simulink subsystem "Out_of_Plane_Model"  (R2025b)
settings: Solver=VariableStepAuto  StartTime=0.0  StopTime=10.0  RelTol=1e-3
undefined symbols (not defined in the file): AeroLiftCff, AeroLongDrgCff, AeroMotoEffctArea, AeroPitchMomentCff, AeroPitchMomentLngth, AeroRltWindAngVect, AeroSideFrcCff, AeroYawMomentCff, aMode, BrkFrntBrkActrBore, BrkFrntBrkActrPrsBpt, BrkFrntBrkPadMeanRadius, BrkFrntBrkTrqTbl, BrkFrntIntrnRadius, BrkFrntKinFricCff, BrkFrntPadNum, BrkFrntShoePinToDrumCntrDst, BrkFrntShoePinToFrcAppDst, BrkFrntShoePinToPadEndAng, BrkFrntShoePinToPadStartAng, BrkFrntStcFricCff, BrkFrntWhlSpdBpt, BrkRearBrkActrBore, BrkRearBrkActrPrsBpt, BrkRearBrkPadMeanRadius, BrkRearBrkTrqTbl, BrkRearIntrnRadius, BrkRearKinFricCff, BrkRearPadNum, BrkRearShoePinToDrumCntrDst, BrkRearShoePinToFrcAppDst, BrkRearShoePinToPadEndAng, BrkRearShoePinToPadStartAng, BrkRearStcFricCff, BrkRearWhlSpdBpt, CpRrVx0, CpRrVy0, CpRrY0, EnvAbsPrs, EnvAirTemp, FrkFrL0, FrmAng0, g, GasCnst, InitFrkLngth, InitMainFrmPitchAng, InitRearArmPitchAng, InitRearCntctPtchLatVel, InitRearCntctPtchLongVel, InitRearCntctPtchZ, InitYawAng, MotoFrmLngth, MotoFrmMass, MotoGrvty, MotoLatOfst, MotoLongOfst, MotoLowrFrntFrkMass, MotoPtchOfst, MotoRearArmLngth, MotoRearArmMass ... (+28)
libraries: sm_lib x309, nesl_utility_internal x158, nesl_utility x7, autolibsharedcoupling x6, vehdynlibtire x6, sharedtransform x4, shared6dof x1, matrix_library x1, vehdynlibeomcommon x1
(part 10 of 10)

== system Out_of_Plane_Model/Chassis, Tires, and Areo/Tire/Front Tire/Linear Front Simscape Tire/Brake model/MW Brake/Brakes/No Brake ==
  BrkPrs : Inport
  Omega : Inport  Port=2
  Ground : Ground
  Terminator : Terminator
  Terminator1 : Terminator
  MyBrk : Outport  VectorParamsAs1DForOutWhenUnconnected=off
  wires:
  BrkPrs/1 -> Terminator/1
  Ground/1 -> MyBrk/1
  Omega/1 -> Terminator1/1

== system Out_of_Plane_Model/Chassis, Tires, and Areo/Tire/Front Tire/Linear Front Simscape Tire/Friction model/External/Calc. part Vertical load & SideSlipAngle/Pythagorean theorem ==
  X : Inport
  Y : Inport  Port=2
  Add2 : Sum
  Math Function : Math  Operator=square  SignedPower=on
  Math Function1 : Math  Operator=square  SignedPower=on
  Sqrt : Sqrt
  sqrt(X^2+Y^2) : Outport  VectorParamsAs1DForOutWhenUnconnected=off
  wires:
  Sqrt/1 -> sqrt(X^2+Y^2)/1
  X/1 -> Math Function/1
  Y/1 -> Math Function1/1
  Math Function/1 -> Add2/1
  Math Function1/1 -> Add2/2
  Add2/1 -> Sqrt/1

== system Out_of_Plane_Model/Chassis, Tires, and Areo/Tire/Front Tire/Linear Front Simscape Tire/Friction model/LinearOld/Calc. part Vertical load & SideSlipAngle/Pythagorean theorem ==
  X : Inport
  Y : Inport  Port=2
  Add2 : Sum
  Math Function : Math  Operator=square  SignedPower=on
  Math Function1 : Math  Operator=square  SignedPower=on
  Sqrt : Sqrt
  sqrt(X^2+Y^2) : Outport  VectorParamsAs1DForOutWhenUnconnected=off
  wires:
  Sqrt/1 -> sqrt(X^2+Y^2)/1
  X/1 -> Math Function/1
  Y/1 -> Math Function1/1
  Math Function/1 -> Add2/1
  Math Function1/1 -> Add2/2
  Add2/1 -> Sqrt/1

== system Out_of_Plane_Model/Chassis, Tires, and Areo/Tire/Front Tire/Linear Front Simscape Tire/Friction model/LinearOld/SlipRatio/Slip Ratio _ Braking ==
  RoadVelocity : Inport
  SlipAngle : Inport  Port=2
  Rot.Velocity : Inport  Port=3
  Add : Sum  Inputs=+-
  Add1 : Sum
  Constant : Constant  Value=1e-5
  Divide : Product  Inputs=**
  Divide1 : Product  Inputs=/*
  Gain : Gain  Gain=pi/180
  Tire radius : Constant  Value=RWhl
  Trigonometric Function : Trigonometry  Operator=cos
  VB : Product  Inputs=**
  Sbb : Outport  VectorParamsAs1DForOutWhenUnconnected=off
  Switch flag : Outport  Port=2  VectorParamsAs1DForOutWhenUnconnected=off
  wires:
  VB/1 -> Add/2
  Rot.Velocity/1 -> VB/2
  Divide1/1 -> Sbb/1
  RoadVelocity/1 -> Divide/1
  SlipAngle/1 -> Gain/1
  Tire radius/1 -> VB/1
  Add/1 -> Switch flag/1, Divide1/2
  Gain/1 -> Trigonometric Function/1
  Trigonometric Function/1 -> Divide/2
  Divide/1 -> Add1/2, Add/1
  Constant/1 -> Add1/1
  Add1/1 -> Divide1/1

== system Out_of_Plane_Model/Chassis, Tires, and Areo/Tire/Front Tire/Linear Front Simscape Tire/Friction model/LinearOld/SlipRatio/Slip Ratio _ Driving ==
  Road velocity : Inport
  SlipAngle : Inport  Port=2
  Rot.Velocity : Inport  Port=3
  Add : Sum  Inputs=+-
  Add1 : Sum
  Constant : Constant  Value=1e-5
  Divide : Product  Inputs=**
  Divide1 : Product  Inputs=*/
  Gain : Gain  Gain=pi/180
  Tire radius : Constant  Value=RWhl
  Trigonometric Function : Trigonometry  Operator=cos
  VB : Product  Inputs=**
  Sbd : Outport  VectorParamsAs1DForOutWhenUnconnected=off
  wires:
  Trigonometric Function/1 -> Divide/2
  Gain/1 -> Trigonometric Function/1
  Divide/1 -> Add/1
  Add/1 -> Divide1/1
  Tire radius/1 -> VB/1
  SlipAngle/1 -> Gain/1
  Road velocity/1 -> Divide/1
  Divide1/1 -> Sbd/1
  Rot.Velocity/1 -> VB/2
  VB/1 -> Add1/1, Add/2
  Add1/1 -> Divide1/2
  Constant/1 -> Add1/2

== system Out_of_Plane_Model/Chassis, Tires, and Areo/Tire/Front Tire/Linear Front Simscape Tire/Simscape/Simscape Multibody Rim&Wheel/Tire_Rim_wth_transient/CPSensor ==
  Bus Creator : BusCreator  Inputs=3
  Bus Creator1 : BusCreator  Inputs=3
  Bus Creator2 : BusCreator  Inputs=3
  Bus Creator3 : BusCreator  Inputs=1
  Origin : Subsystem
  PS-Simulink Converter{1..10} (10 alike) : nesl_utility_internal/PS-Simulink Converter  PhysicalDomain=network_engine_domain  SubClassName=ps_output  LeftPortType=input  RightPortType=output  PseudoPeriodic=off  Frequencies=[]  VectorFormat=1-D array  Unit=inherit  AffineConversion=off
  Transform Sensor : sm_lib/Frames and Transforms/Transform Sensor  MeasurementFrame=NonRotatingBase  RotationSequence=XYX  SenseAngle=off  SenseAxis=off  SenseQ=off  SenseR=off  SenseRotationSequence=off  SenseOmegaX=off  SenseOmegaY=off  SenseOmegaZ=on  SenseOmega=off  SenseQDot=off  SenseRDot=off  SenseRotationSequenceDot=off  SenseAlphaX=off  SenseAlphaY=off  SenseAlphaZ=off  SenseAlpha=off  SenseQDDot=off  SenseRDDot=off  SenseX=on  SenseY=on  SenseZ=on  SenseXYZ=off  SenseRad=off  SenseAzim=off  SenseDist=off  SenseInc=off  SenseXDot=on  SenseYDot=on  SenseZDot=on  SenseXYZDot=off  SenseRadDot=off  SenseAzimDot=off  SenseDistDot=off  SenseIncDot=off  SenseXDDot=on  SenseYDDot=on  SenseZDDot=on  SenseXYZDDot=off  SenseRadDDot=off  SenseAzimDDot=off  SenseDistDDot=off  SenseIncDDot=off
  F : PMIOPort  Side=Right
  WhlCpX : Outport
  WhlCpY : Outport  Port=2
  WhlCpZ : Outport  Port=3
  WhlCpVPsi : Outport  Port=4
  wires:
  PS-Simulink Converter7/1 -> Bus Creator/2  "WhlCpVx"
  PS-Simulink Converter6/1 -> Bus Creator2/3  "WhlCpPy"
  PS-Simulink Converter8/1 -> Bus Creator1/3  "WhlCpPz"
  PS-Simulink Converter9/1 -> Bus Creator1/2  "WhlCpVz"
  PS-Simulink Converter5/1 -> Bus Creator/3  "WhlCpPx"
  PS-Simulink Converter3/1 -> Bus Creator1/1  "WhlCpAz"
  PS-Simulink Converter4/1 -> Bus Creator2/2  "WhlCpVy"
  Bus Creator2/1 -> WhlCpY/1  "WhlCpY"
  PS-Simulink Converter2/1 -> Bus Creator/1  "WhlCpAx"
  PS-Simulink Converter1/1 -> Bus Creator2/1  "WhlCpAy"
  Bus Creator/1 -> WhlCpX/1  "WhlCpX"
  Bus Creator1/1 -> WhlCpZ/1  "WhlCpZ"
  PS-Simulink Converter10/1 -> Bus Creator3/1  "WhlCpVPsi"
  Bus Creator3/1 -> WhlCpVPsi/1  "WhlCpPsi"
  connections:
  Transform Sensor/RConn10 -- PS-Simulink Converter1/LConn1
  Transform Sensor/RConn8 -- PS-Simulink Converter9/LConn1
  Transform Sensor/RConn3 -- PS-Simulink Converter5/LConn1
  Transform Sensor/RConn11 -- PS-Simulink Converter3/LConn1
  Transform Sensor/RConn9 -- PS-Simulink Converter2/LConn1
  Transform Sensor/RConn6 -- PS-Simulink Converter7/LConn1
  Transform Sensor/RConn7 -- PS-Simulink Converter4/LConn1
  Transform Sensor/RConn5 -- PS-Simulink Converter8/LConn1
  Transform Sensor/RConn4 -- PS-Simulink Converter6/LConn1
  PS-Simulink Converter10/LConn1 -- Transform Sensor/RConn2
  F/RConn1 -- Transform Sensor/RConn1
  Origin/RConn1 -- Transform Sensor/LConn1

== system Out_of_Plane_Model/Chassis, Tires, and Areo/Tire/Front Tire/Linear Front Simscape Tire/Simscape/Simscape Multibody Rim&Wheel/Tire_Rim_wth_transient/Pitch dof ==
  Rigid Transform : sm_lib/Frames and Transforms/Rigid Transform  RotationMethod=StandardAxis  FollAlignAxisA=+X  BaseAlignAxisA=+Y  FollAlignAxisB=+Y  BaseAlignAxisB=+Z  RotationStandardAxis=+X  RotationAngle=-pi/2  RotationAngleUnits=rad  RotationArbitraryAxis=[0 0 1]  RotationSequenceAxes=FollowerAxes  RotationSequence=XYX  RotationSequenceAngles=[0 0 0]  RotationSequenceAnglesUnits=deg  RotationMatrix=[1 0 0; 0 1 0; 0 0 1]  Quaternion=[1 0 0 0]  TranslationMethod=None  TranslationCartesianOffset=[0 0 0]  TranslationCartesianOffsetUnits=m  TranslationStandardAxis=+X  TranslationStandardOffset=0  TranslationStandardOffsetUnits=m  TranslationROffset=0  TranslationROffsetUnits=m  TranslationThetaOffset=0  TranslationThetaOffsetUnits=deg  TranslationZOffset=0  TranslationZOffsetUnits=m
  Rigid Transform1 : sm_lib/Frames and Transforms/Rigid Transform  RotationMethod=StandardAxis  FollAlignAxisA=+X  BaseAlignAxisA=+Y  FollAlignAxisB=+Y  BaseAlignAxisB=+Z  RotationStandardAxis=+X  RotationAngle=pi/2  RotationAngleUnits=rad  RotationArbitraryAxis=[0 0 1]  RotationSequenceAxes=FollowerAxes  RotationSequence=XYX  RotationSequenceAngles=[0 0 0]  RotationSequenceAnglesUnits=deg  RotationMatrix=[1 0 0; 0 1 0; 0 0 1]  Quaternion=[1 0 0 0]  TranslationMethod=None  TranslationCartesianOffset=[0 0 0]  TranslationCartesianOffsetUnits=m  TranslationStandardAxis=+X  TranslationStandardOffset=0  TranslationStandardOffsetUnits=m  TranslationROffset=0  TranslationROffsetUnits=m  TranslationThetaOffset=0  TranslationThetaOffsetUnits=deg  TranslationZOffset=0  TranslationZOffsetUnits=m
  rev : sm_lib/Joints/Revolute Joint  JointMode=Normal  CompositeWrenchDir=FollowerOnBase  CompositeWrenchFrame=BaseFrame  SenseConstraintForce=off  SenseConstraintTorque=off  SenseTotalForce=off  SenseTotalTorque=off  PositionTargetSpecify=off  PositionTargetPriority=High  PositionTargetValue=0  PositionTargetValueUnits=deg  VelocityTargetSpecify=off  VelocityTargetPriority=High  VelocityTargetValue=0  VelocityTargetValueUnits=rad/s  EquilibriumPosition=0  EquilibriumPositionUnits=deg  SpringStiffness=0  SpringStiffnessUnits=N*m/deg  DampingCoefficient=0  DampingCoefficientUnits=N*m/(rad/s)  LowerLimitSpecify=off  LowerLimitBound=-90  LowerLimitBoundUnits=deg  LowerLimitStiffness=1e4  LowerLimitStiffnessUnits=N*m/deg  LowerLimitDamping=10  LowerLimitDampingUnits=N*m/(deg/s)  LowerLimitTransitionRegionWidth=0.1  LowerLimitTransitionRegionWidthUnits=deg  UpperLimitSpecify=off  UpperLimitBound=90  UpperLimitBoundUnits=deg  UpperLimitStiffness=1e4  UpperLimitStiffnessUnits=N*m/deg  UpperLimitDamping=10  UpperLimitDampingUnits=N*m/(deg/s)  UpperLimitTransitionRegionWidth=0.1  UpperLimitTransitionRegionWidthUnits=deg  TorqueActuationMode=NoTorque  MotionActuationMode=ComputedMotion  SensePosition=off  SenseVelocity=off  SenseAcceleration=off  SenseTorqueForce=off  SenseLowerLimitTorqueForce=off  SenseUpperLimitTorqueForce=off
  B : PMIOPort  Side=Left
  F : PMIOPort  Port=2  Side=Right
  connections:
  rev/RConn1 -- Rigid Transform1/LConn1
  Rigid Transform1/RConn1 -- F/RConn1
  Rigid Transform/RConn1 -- rev/LConn1
  Rigid Transform/LConn1 -- B/RConn1

== system Out_of_Plane_Model/Chassis, Tires, and Areo/Tire/Front Tire/Linear Front Simscape Tire/Simscape/Simscape Multibody Rim&Wheel/Tire_Rim_wth_transient/Roll dof ==
  Bus Creator : BusCreator  Inputs=3
  PS-Simulink Converter : nesl_utility_internal/PS-Simulink Converter  PhysicalDomain=network_engine_domain  SubClassName=ps_output  LeftPortType=input  RightPortType=output  PseudoPeriodic=off  Frequencies=[]  VectorFormat=1-D array  Unit=inherit  AffineConversion=off
  PS-Simulink Converter1 : nesl_utility_internal/PS-Simulink Converter  PhysicalDomain=network_engine_domain  SubClassName=ps_output  LeftPortType=input  RightPortType=output  PseudoPeriodic=off  Frequencies=[]  VectorFormat=1-D array  Unit=inherit  AffineConversion=off
  PS-Simulink Converter2 : nesl_utility_internal/PS-Simulink Converter  PhysicalDomain=network_engine_domain  SubClassName=ps_output  LeftPortType=input  RightPortType=output  PseudoPeriodic=off  Frequencies=[]  VectorFormat=1-D array  Unit=inherit  AffineConversion=off
  Rev : sm_lib/Joints/Revolute Joint  JointMode=Normal  CompositeWrenchDir=FollowerOnBase  CompositeWrenchFrame=BaseFrame  SenseConstraintForce=off  SenseConstraintTorque=off  SenseTotalForce=off  SenseTotalTorque=off  PositionTargetSpecify=off  PositionTargetPriority=High  PositionTargetValue=0  PositionTargetValueUnits=deg  VelocityTargetSpecify=off  VelocityTargetPriority=High  VelocityTargetValue=0  VelocityTargetValueUnits=rad/s  EquilibriumPosition=0  EquilibriumPositionUnits=rad  SpringStiffness=0  SpringStiffnessUnits=N*m/rad  DampingCoefficient=0  DampingCoefficientUnits=N*m/(rad/s)  LowerLimitSpecify=off  LowerLimitBound=-90  LowerLimitBoundUnits=deg  LowerLimitStiffness=1e4  LowerLimitStiffnessUnits=N*m/deg  LowerLimitDamping=10  LowerLimitDampingUnits=N*m/(deg/s)  LowerLimitTransitionRegionWidth=0.1  LowerLimitTransitionRegionWidthUnits=deg  UpperLimitSpecify=off  UpperLimitBound=90  UpperLimitBoundUnits=deg  UpperLimitStiffness=1e4  UpperLimitStiffnessUnits=N*m/deg  UpperLimitDamping=10  UpperLimitDampingUnits=N*m/(deg/s)  UpperLimitTransitionRegionWidth=0.1  UpperLimitTransitionRegionWidthUnits=deg  TorqueActuationMode=NoTorque  MotionActuationMode=ComputedMotion  SensePosition=on  SenseVelocity=on  SenseAcceleration=on  SenseTorqueForce=off  SenseLowerLimitTorqueForce=off  SenseUpperLimitTorqueForce=off
  Unary Minus : UnaryMinus
  Unary Minus1 : UnaryMinus
  Unary Minus2 : UnaryMinus
  Y_-pi/2 : sm_lib/Frames and Transforms/Rigid Transform  RotationMethod=StandardAxis  FollAlignAxisA=+X  BaseAlignAxisA=+Y  FollAlignAxisB=+Y  BaseAlignAxisB=+Z  RotationStandardAxis=+Y  RotationAngle=-pi/2  RotationAngleUnits=rad  RotationArbitraryAxis=[0 0 1]  RotationSequenceAxes=FollowerAxes  RotationSequence=XYX  RotationSequenceAngles=[0 0 0]  RotationSequenceAnglesUnits=deg  RotationMatrix=[1 0 0; 0 1 0; 0 0 1]  Quaternion=[1 0 0 0]  TranslationMethod=None  TranslationCartesianOffset=[0 0 0]  TranslationCartesianOffsetUnits=m  TranslationStandardAxis=+Z  TranslationStandardOffset=0  TranslationStandardOffsetUnits=m  TranslationROffset=0  TranslationROffsetUnits=m  TranslationThetaOffset=0  TranslationThetaOffsetUnits=deg  TranslationZOffset=0  TranslationZOffsetUnits=m
  Y_pi/2 : sm_lib/Frames and Transforms/Rigid Transform  RotationMethod=StandardAxis  FollAlignAxisA=+X  BaseAlignAxisA=+Y  FollAlignAxisB=+Y  BaseAlignAxisB=+Z  RotationStandardAxis=+Y  RotationAngle=pi/2  RotationAngleUnits=rad  RotationArbitraryAxis=[0 0 1]  RotationSequenceAxes=FollowerAxes  RotationSequence=XYX  RotationSequenceAngles=[0 0 0]  RotationSequenceAnglesUnits=deg  RotationMatrix=[1 0 0; 0 1 0; 0 0 1]  Quaternion=[1 0 0 0]  TranslationMethod=None  TranslationCartesianOffset=[0 0 0]  TranslationCartesianOffsetUnits=m  TranslationStandardAxis=+Z  TranslationStandardOffset=0  TranslationStandardOffsetUnits=m  TranslationROffset=0  TranslationROffsetUnits=m  TranslationThetaOffset=0  TranslationThetaOffsetUnits=deg  TranslationZOffset=0  TranslationZOffsetUnits=m
  B : PMIOPort  Side=Left
  F : PMIOPort  Port=2  Side=Right
  A,V,P_WhlRoll : Outport
  wires:
  PS-Simulink Converter/1 -> Unary Minus/1  "WhlPRoll"
  PS-Simulink Converter1/1 -> Unary Minus1/1  "WhlVRoll"
  PS-Simulink Converter2/1 -> Unary Minus2/1  "WhlARoll"
  Bus Creator/1 -> A,V,P_WhlRoll/1  "WhlRrCpX"
  Unary Minus/1 -> Bus Creator/3  "WhlPRoll"
  Unary Minus1/1 -> Bus Creator/2  "WhlVRoll"
  Unary Minus2/1 -> Bus Creator/1  "WhlARoll"
  connections:
  Rev/RConn3 -- PS-Simulink Converter1/LConn1
  PS-Simulink Converter2/LConn1 -- Rev/RConn4
  PS-Simulink Converter/LConn1 -- Rev/RConn2
  Y_-pi/2/RConn1 -- F/RConn1
  Y_pi/2/RConn1 -- Rev/LConn1
  Y_-pi/2/LConn1 -- Rev/RConn1
  Y_pi/2/LConn1 -- B/RConn1

== system Out_of_Plane_Model/Chassis, Tires, and Areo/Tire/Front Tire/Linear Front Simscape Tire/Simscape/Simscape Multibody Rim&Wheel/Tire_Rim_wth_transient/dofPitch ==
  HubJoint : sm_lib/Joints/Revolute Joint  JointMode=Normal  CompositeWrenchDir=FollowerOnBase  CompositeWrenchFrame=BaseFrame  SenseConstraintForce=off  SenseConstraintTorque=off  SenseTotalForce=off  SenseTotalTorque=off  PositionTargetSpecify=off  PositionTargetPriority=High  PositionTargetValue=0  PositionTargetValueUnits=deg  VelocityTargetSpecify=on  VelocityTargetPriority=High  VelocityTargetValue=omegao  VelocityTargetValueUnits=rad/s  EquilibriumPosition=0  EquilibriumPositionUnits=deg  SpringStiffness=0  SpringStiffnessUnits=N*m/deg  DampingCoefficient=0  DampingCoefficientUnits=N*m/(rad/s)  LowerLimitSpecify=off  LowerLimitBound=-90  LowerLimitBoundUnits=deg  LowerLimitStiffness=1e4  LowerLimitStiffnessUnits=N*m/deg  LowerLimitDamping=10  LowerLimitDampingUnits=N*m/(deg/s)  LowerLimitTransitionRegionWidth=0.1  LowerLimitTransitionRegionWidthUnits=deg  UpperLimitSpecify=off  UpperLimitBound=90  UpperLimitBoundUnits=deg  UpperLimitStiffness=1e4  UpperLimitStiffnessUnits=N*m/deg  UpperLimitDamping=10  UpperLimitDampingUnits=N*m/(deg/s)  UpperLimitTransitionRegionWidth=0.1  UpperLimitTransitionRegionWidthUnits=deg  TorqueActuationMode=NoTorque  MotionActuationMode=ComputedMotion  SensePosition=off  SenseVelocity=on  SenseAcceleration=on  SenseTorqueForce=off  SenseLowerLimitTorqueForce=off  SenseUpperLimitTorqueForce=off
  PS-Simulink Converter : nesl_utility_internal/PS-Simulink Converter  PhysicalDomain=network_engine_domain  SubClassName=ps_output  LeftPortType=input  RightPortType=output  PseudoPeriodic=off  Frequencies=[]  VectorFormat=1-D array  Unit=inherit  AffineConversion=off
  PS-Simulink Converter1 : nesl_utility_internal/PS-Simulink Converter  PhysicalDomain=network_engine_domain  SubClassName=ps_output  LeftPortType=input  RightPortType=output  PseudoPeriodic=off  Frequencies=[]  VectorFormat=1-D array  Unit=inherit  AffineConversion=off
  Rigid Transform : sm_lib/Frames and Transforms/Rigid Transform  RotationMethod=StandardAxis  FollAlignAxisA=+X  BaseAlignAxisA=+Y  FollAlignAxisB=+Y  BaseAlignAxisB=+Z  RotationStandardAxis=+X  RotationAngle=-pi/2  RotationAngleUnits=rad  RotationArbitraryAxis=[0 0 1]  RotationSequenceAxes=FollowerAxes  RotationSequence=XYX  RotationSequenceAngles=[0 0 0]  RotationSequenceAnglesUnits=deg  RotationMatrix=[1 0 0; 0 1 0; 0 0 1]  Quaternion=[1 0 0 0]  TranslationMethod=None  TranslationCartesianOffset=[0 0 0]  TranslationCartesianOffsetUnits=m  TranslationStandardAxis=+X  TranslationStandardOffset=0  TranslationStandardOffsetUnits=m  TranslationROffset=0  TranslationROffsetUnits=m  TranslationThetaOffset=0  TranslationThetaOffsetUnits=deg  TranslationZOffset=0  TranslationZOffsetUnits=m
  Rigid Transform1 : sm_lib/Frames and Transforms/Rigid Transform  RotationMethod=StandardAxis  FollAlignAxisA=+X  BaseAlignAxisA=+Y  FollAlignAxisB=+Y  BaseAlignAxisB=+Z  RotationStandardAxis=+X  RotationAngle=pi/2  RotationAngleUnits=rad  RotationArbitraryAxis=[0 0 1]  RotationSequenceAxes=FollowerAxes  RotationSequence=XYX  RotationSequenceAngles=[0 0 0]  RotationSequenceAnglesUnits=deg  RotationMatrix=[1 0 0; 0 1 0; 0 0 1]  Quaternion=[1 0 0 0]  TranslationMethod=None  TranslationCartesianOffset=[0 0 0]  TranslationCartesianOffsetUnits=m  TranslationStandardAxis=+X  TranslationStandardOffset=0  TranslationStandardOffsetUnits=m  TranslationROffset=0  TranslationROffsetUnits=m  TranslationThetaOffset=0  TranslationThetaOffsetUnits=deg  TranslationZOffset=0  TranslationZOffsetUnits=m
  B : PMIOPort  Side=Left
  F : PMIOPort  Port=2  Side=Right
  omega : Outport
  omegadot : Outport  Port=2
  wires:
  PS-Simulink Converter/1 -> omega/1
  PS-Simulink Converter1/1 -> omegadot/1
  connections:
  Rigid Transform/LConn1 -- B/RConn1
  Rigid Transform/RConn1 -- HubJoint/LConn1
  Rigid Transform1/RConn1 -- F/RConn1
  HubJoint/RConn1 -- Rigid Transform1/LConn1
  PS-Simulink Converter/LConn1 -- HubJoint/RConn2
  PS-Simulink Converter1/LConn1 -- HubJoint/RConn3

== system Out_of_Plane_Model/Chassis, Tires, and Areo/Tire/Rear Tire/Linear Rear Simscape Tire/Brake model/MW Brake/Brakes/Disk Brake ==
  BrkPrs : Inport
  Omega : Inport  Port=2
  Disk Brake : autolibsharedcoupling/Rotational Brake  BrakeType=Disc  rotType=No inertia  extInfo=off  Iyy=1  br=1e-3  omegao=0  mu_static=BrkRearStcFricCff  mu_kinetic=BrkRearKinFricCff  disk_abore=BrkRearBrkActrBore  Rm=BrkRearBrkPadMeanRadius  num_pads=BrkRearPadNum  drum_abore=BrkRearBrkActrBore  drum_a=BrkRearShoePinToDrumCntrDst  drum_c=BrkRearShoePinToFrcAppDst  drum_r=BrkRearIntrnRadius  drum_theta1=BrkRearShoePinToPadStartAng  drum_theta2=BrkRearShoePinToPadEndAng  brake_p_bpt=BrkReartBrkActrPrsBpt  brake_n_bpt=BrkRearWhlSpdBpt  f_brake_t=BrkRearBrkTrqTbl  aMode=2
      settings: LibrarySourceBlock=vehdynlibbrake/Disc Brake
  MyBrk : Outport  VectorParamsAs1DForOutWhenUnconnected=off
  wires:
  BrkPrs/1 -> Disk Brake/1
  Omega/1 -> Disk Brake/2
  Disk Brake/1 -> MyBrk/1

== system Out_of_Plane_Model/Chassis, Tires, and Areo/Tire/Rear Tire/Linear Rear Simscape Tire/Brake model/MW Brake/Brakes/Drum Brake ==
  BrkPrs : Inport
  Omega : Inport  Port=2
  Drum Brake : autolibsharedcoupling/Rotational Brake  BrakeType=Drum  rotType=No inertia  extInfo=off  Iyy=1  br=1e-3  omegao=0  mu_static=BrkRearStcFricCff  mu_kinetic=BrkRearKinFricCff  disk_abore=BrkRearBrkActrBore  Rm=BrkRearBrkPadMeanRadius  num_pads=BrkRearPadNum  drum_abore=BrkRearBrkActrBore  drum_a=BrkRearShoePinToDrumCntrDst  drum_c=BrkRearShoePinToFrcAppDst  drum_r=BrkRearIntrnRadius  drum_theta1=BrkRearShoePinToPadStartAng  drum_theta2=BrkRearShoePinToPadEndAng  brake_p_bpt=BrkReartBrkActrPrsBpt  brake_n_bpt=BrkRearWhlSpdBpt  f_brake_t=BrkRearBrkTrqTbl  aMode=2
      settings: LibrarySourceBlock=vehdynlibbrake/Disc Brake
  MyBrk : Outport  VectorParamsAs1DForOutWhenUnconnected=off
  wires:
  Drum Brake/1 -> MyBrk/1
  Omega/1 -> Drum Brake/2
  BrkPrs/1 -> Drum Brake/1

== system Out_of_Plane_Model/Chassis, Tires, and Areo/Tire/Rear Tire/Linear Rear Simscape Tire/Brake model/MW Brake/Brakes/Mapped Brake ==
  BrkPrs : Inport
  Omega : Inport  Port=2
  Mapped Brake : autolibsharedcoupling/Rotational Brake  BrakeType=Mapped  rotType=No inertia  extInfo=off  Iyy=1  br=1e-3  omegao=0  mu_static=BrkRearStcFricCff  mu_kinetic=BrkRearKinFricCff  disk_abore=BrkRearBrkActrBore  Rm=BrkRearBrkPadMeanRadius  num_pads=BrkRearPadNum  drum_abore=BrkRearBrkActrBore  drum_a=BrkRearShoePinToDrumCntrDst  drum_c=BrkRearShoePinToFrcAppDst  drum_r=BrkRearIntrnRadius  drum_theta1=BrkRearShoePinToPadStartAng  drum_theta2=BrkRearShoePinToPadEndAng  brake_p_bpt=BrkReartBrkActrPrsBpt  brake_n_bpt=BrkRearWhlSpdBpt  f_brake_t=BrkRearBrkTrqTbl  aMode=2
      settings: LibrarySourceBlock=vehdynlibbrake/Disc Brake
  MyBrk : Outport  VectorParamsAs1DForOutWhenUnconnected=off
  wires:
  Omega/1 -> Mapped Brake/2
  Mapped Brake/1 -> MyBrk/1
  BrkPrs/1 -> Mapped Brake/1

== system Out_of_Plane_Model/Chassis, Tires, and Areo/Tire/Rear Tire/Linear Rear Simscape Tire/Brake model/MW Brake/Brakes/No Brake ==
  BrkPrs : Inport
  Omega : Inport  Port=2
  Ground : Ground
  Terminator : Terminator
  Terminator1 : Terminator
  MyBrk : Outport  VectorParamsAs1DForOutWhenUnconnected=off
  wires:
  BrkPrs/1 -> Terminator/1
  Ground/1 -> MyBrk/1
  Omega/1 -> Terminator1/1

== system Out_of_Plane_Model/Chassis, Tires, and Areo/Tire/Rear Tire/Linear Rear Simscape Tire/Friction model/External/Calc. part Vertical load & SideSlipAngle/Pythagorean theorem ==
  X : Inport
  Y : Inport  Port=2
  Add2 : Sum
  Math Function : Math  Operator=square  SignedPower=on
  Math Function1 : Math  Operator=square  SignedPower=on
  Sqrt : Sqrt
  sqrt(X^2+Y^2) : Outport  VectorParamsAs1DForOutWhenUnconnected=off
  wires:
  Sqrt/1 -> sqrt(X^2+Y^2)/1
  X/1 -> Math Function/1
  Y/1 -> Math Function1/1
  Math Function/1 -> Add2/1
  Math Function1/1 -> Add2/2
  Add2/1 -> Sqrt/1

== system Out_of_Plane_Model/Chassis, Tires, and Areo/Tire/Rear Tire/Linear Rear Simscape Tire/Friction model/LinearOld/Calc. part Vertical load & SideSlipAngle/Pythagorean theorem ==
  X : Inport
  Y : Inport  Port=2
  Add2 : Sum
  Math Function : Math  Operator=square  SignedPower=on
  Math Function1 : Math  Operator=square  SignedPower=on
  Sqrt : Sqrt
  sqrt(X^2+Y^2) : Outport  VectorParamsAs1DForOutWhenUnconnected=off
  wires:
  Sqrt/1 -> sqrt(X^2+Y^2)/1
  X/1 -> Math Function/1
  Y/1 -> Math Function1/1
  Math Function/1 -> Add2/1
  Math Function1/1 -> Add2/2
  Add2/1 -> Sqrt/1

== system Out_of_Plane_Model/Chassis, Tires, and Areo/Tire/Rear Tire/Linear Rear Simscape Tire/Friction model/LinearOld/SlipRatio/Slip Ratio _ Braking ==
  RoadVelocity : Inport
  SlipAngle : Inport  Port=2
  Rot.Velocity : Inport  Port=3
  Add : Sum  Inputs=+-
  Add1 : Sum
  Constant : Constant  Value=1e-5
  Divide : Product  Inputs=**
  Divide1 : Product  Inputs=/*
  Gain : Gain  Gain=pi/180
  Tire radius : Constant  Value=RWhl
  Trigonometric Function : Trigonometry  Operator=cos
  VB : Product  Inputs=**
  Sbb : Outport  VectorParamsAs1DForOutWhenUnconnected=off
  Switch flag : Outport  Port=2  VectorParamsAs1DForOutWhenUnconnected=off
  wires:
  VB/1 -> Add/2
  Rot.Velocity/1 -> VB/2
  Divide1/1 -> Sbb/1
  RoadVelocity/1 -> Divide/1
  SlipAngle/1 -> Gain/1
  Tire radius/1 -> VB/1
  Add/1 -> Switch flag/1, Divide1/2
  Gain/1 -> Trigonometric Function/1
  Trigonometric Function/1 -> Divide/2
  Divide/1 -> Add1/2, Add/1
  Constant/1 -> Add1/1
  Add1/1 -> Divide1/1

== system Out_of_Plane_Model/Chassis, Tires, and Areo/Tire/Rear Tire/Linear Rear Simscape Tire/Friction model/LinearOld/SlipRatio/Slip Ratio _ Driving ==
  Road velocity : Inport
  SlipAngle : Inport  Port=2
  Rot.Velocity : Inport  Port=3
  Add : Sum  Inputs=+-
  Add1 : Sum
  Constant : Constant  Value=1e-5
  Divide : Product  Inputs=**
  Divide1 : Product  Inputs=*/
  Gain : Gain  Gain=pi/180
  Tire radius : Constant  Value=RWhl
  Trigonometric Function : Trigonometry  Operator=cos
  VB : Product  Inputs=**
  Sbd : Outport  VectorParamsAs1DForOutWhenUnconnected=off
  wires:
  Trigonometric Function/1 -> Divide/2
  Gain/1 -> Trigonometric Function/1
  Divide/1 -> Add/1
  Add/1 -> Divide1/1
  Tire radius/1 -> VB/1
  SlipAngle/1 -> Gain/1
  Road velocity/1 -> Divide/1
  Divide1/1 -> Sbd/1
  Rot.Velocity/1 -> VB/2
  VB/1 -> Add1/1, Add/2
  Add1/1 -> Divide1/2
  Constant/1 -> Add1/2

== system Out_of_Plane_Model/Chassis, Tires, and Areo/Tire/Rear Tire/Linear Rear Simscape Tire/Simscape/Simscape Multibody Rim&Wheel/Tire_Rim_wth_transient/CPSensor ==
  Bus Creator : BusCreator  Inputs=3
  Bus Creator1 : BusCreator  Inputs=3
  Bus Creator2 : BusCreator  Inputs=3
  Bus Creator3 : BusCreator  Inputs=1
  Origin : Subsystem
  PS-Simulink Converter{1..10} (10 alike) : nesl_utility_internal/PS-Simulink Converter  PhysicalDomain=network_engine_domain  SubClassName=ps_output  LeftPortType=input  RightPortType=output  PseudoPeriodic=off  Frequencies=[]  VectorFormat=1-D array  Unit=inherit  AffineConversion=off
  Transform Sensor : sm_lib/Frames and Transforms/Transform Sensor  MeasurementFrame=NonRotatingBase  RotationSequence=XYX  SenseAngle=off  SenseAxis=off  SenseQ=off  SenseR=off  SenseRotationSequence=off  SenseOmegaX=off  SenseOmegaY=off  SenseOmegaZ=on  SenseOmega=off  SenseQDot=off  SenseRDot=off  SenseRotationSequenceDot=off  SenseAlphaX=off  SenseAlphaY=off  SenseAlphaZ=off  SenseAlpha=off  SenseQDDot=off  SenseRDDot=off  SenseX=on  SenseY=on  SenseZ=on  SenseXYZ=off  SenseRad=off  SenseAzim=off  SenseDist=off  SenseInc=off  SenseXDot=on  SenseYDot=on  SenseZDot=on  SenseXYZDot=off  SenseRadDot=off  SenseAzimDot=off  SenseDistDot=off  SenseIncDot=off  SenseXDDot=on  SenseYDDot=on  SenseZDDot=on  SenseXYZDDot=off  SenseRadDDot=off  SenseAzimDDot=off  SenseDistDDot=off  SenseIncDDot=off
  F : PMIOPort  Side=Right
  WhlCpX : Outport
  WhlCpY : Outport  Port=2
  WhlCpZ : Outport  Port=3
  WhlCpVPsi : Outport  Port=4
  wires:
  PS-Simulink Converter7/1 -> Bus Creator/2  "WhlCpVx"
  PS-Simulink Converter6/1 -> Bus Creator2/3  "WhlCpPy"
  PS-Simulink Converter8/1 -> Bus Creator1/3  "WhlCpPz"
  PS-Simulink Converter9/1 -> Bus Creator1/2  "WhlCpVz"
  PS-Simulink Converter5/1 -> Bus Creator/3  "WhlCpPx"
  PS-Simulink Converter3/1 -> Bus Creator1/1  "WhlCpAz"
  PS-Simulink Converter4/1 -> Bus Creator2/2  "WhlCpVy"
  Bus Creator2/1 -> WhlCpY/1  "WhlCpY"
  PS-Simulink Converter2/1 -> Bus Creator/1  "WhlCpAx"
  PS-Simulink Converter1/1 -> Bus Creator2/1  "WhlCpAy"
  Bus Creator/1 -> WhlCpX/1  "WhlCpX"
  Bus Creator1/1 -> WhlCpZ/1  "WhlCpZ"
  PS-Simulink Converter10/1 -> Bus Creator3/1  "WhlCpVPsi"
  Bus Creator3/1 -> WhlCpVPsi/1  "WhlCpPsi"
  connections:
  Transform Sensor/RConn10 -- PS-Simulink Converter1/LConn1
  Transform Sensor/RConn8 -- PS-Simulink Converter9/LConn1
  Transform Sensor/RConn3 -- PS-Simulink Converter5/LConn1
  Transform Sensor/RConn11 -- PS-Simulink Converter3/LConn1
  Transform Sensor/RConn9 -- PS-Simulink Converter2/LConn1
  Transform Sensor/RConn6 -- PS-Simulink Converter7/LConn1
  Transform Sensor/RConn7 -- PS-Simulink Converter4/LConn1
  Transform Sensor/RConn5 -- PS-Simulink Converter8/LConn1
  Transform Sensor/RConn4 -- PS-Simulink Converter6/LConn1
  PS-Simulink Converter10/LConn1 -- Transform Sensor/RConn2
  F/RConn1 -- Transform Sensor/RConn1
  Origin/RConn1 -- Transform Sensor/LConn1

== system Out_of_Plane_Model/Chassis, Tires, and Areo/Tire/Rear Tire/Linear Rear Simscape Tire/Simscape/Simscape Multibody Rim&Wheel/Tire_Rim_wth_transient/Pitch dof ==
  Rigid Transform : sm_lib/Frames and Transforms/Rigid Transform  RotationMethod=StandardAxis  FollAlignAxisA=+X  BaseAlignAxisA=+Y  FollAlignAxisB=+Y  BaseAlignAxisB=+Z  RotationStandardAxis=+X  RotationAngle=-pi/2  RotationAngleUnits=rad  RotationArbitraryAxis=[0 0 1]  RotationSequenceAxes=FollowerAxes  RotationSequence=XYX  RotationSequenceAngles=[0 0 0]  RotationSequenceAnglesUnits=deg  RotationMatrix=[1 0 0; 0 1 0; 0 0 1]  Quaternion=[1 0 0 0]  TranslationMethod=None  TranslationCartesianOffset=[0 0 0]  TranslationCartesianOffsetUnits=m  TranslationStandardAxis=+X  TranslationStandardOffset=0  TranslationStandardOffsetUnits=m  TranslationROffset=0  TranslationROffsetUnits=m  TranslationThetaOffset=0  TranslationThetaOffsetUnits=deg  TranslationZOffset=0  TranslationZOffsetUnits=m
  Rigid Transform1 : sm_lib/Frames and Transforms/Rigid Transform  RotationMethod=StandardAxis  FollAlignAxisA=+X  BaseAlignAxisA=+Y  FollAlignAxisB=+Y  BaseAlignAxisB=+Z  RotationStandardAxis=+X  RotationAngle=pi/2  RotationAngleUnits=rad  RotationArbitraryAxis=[0 0 1]  RotationSequenceAxes=FollowerAxes  RotationSequence=XYX  RotationSequenceAngles=[0 0 0]  RotationSequenceAnglesUnits=deg  RotationMatrix=[1 0 0; 0 1 0; 0 0 1]  Quaternion=[1 0 0 0]  TranslationMethod=None  TranslationCartesianOffset=[0 0 0]  TranslationCartesianOffsetUnits=m  TranslationStandardAxis=+X  TranslationStandardOffset=0  TranslationStandardOffsetUnits=m  TranslationROffset=0  TranslationROffsetUnits=m  TranslationThetaOffset=0  TranslationThetaOffsetUnits=deg  TranslationZOffset=0  TranslationZOffsetUnits=m
  rev : sm_lib/Joints/Revolute Joint  JointMode=Normal  CompositeWrenchDir=FollowerOnBase  CompositeWrenchFrame=BaseFrame  SenseConstraintForce=off  SenseConstraintTorque=off  SenseTotalForce=off  SenseTotalTorque=off  PositionTargetSpecify=off  PositionTargetPriority=High  PositionTargetValue=0  PositionTargetValueUnits=deg  VelocityTargetSpecify=off  VelocityTargetPriority=High  VelocityTargetValue=0  VelocityTargetValueUnits=rad/s  EquilibriumPosition=0  EquilibriumPositionUnits=deg  SpringStiffness=0  SpringStiffnessUnits=N*m/deg  DampingCoefficient=0  DampingCoefficientUnits=N*m/(rad/s)  LowerLimitSpecify=off  LowerLimitBound=-90  LowerLimitBoundUnits=deg  LowerLimitStiffness=1e4  LowerLimitStiffnessUnits=N*m/deg  LowerLimitDamping=10  LowerLimitDampingUnits=N*m/(deg/s)  LowerLimitTransitionRegionWidth=0.1  LowerLimitTransitionRegionWidthUnits=deg  UpperLimitSpecify=off  UpperLimitBound=90  UpperLimitBoundUnits=deg  UpperLimitStiffness=1e4  UpperLimitStiffnessUnits=N*m/deg  UpperLimitDamping=10  UpperLimitDampingUnits=N*m/(deg/s)  UpperLimitTransitionRegionWidth=0.1  UpperLimitTransitionRegionWidthUnits=deg  TorqueActuationMode=NoTorque  MotionActuationMode=ComputedMotion  SensePosition=off  SenseVelocity=off  SenseAcceleration=off  SenseTorqueForce=off  SenseLowerLimitTorqueForce=off  SenseUpperLimitTorqueForce=off
  B : PMIOPort  Side=Left
  F : PMIOPort  Port=2  Side=Right
  connections:
  rev/RConn1 -- Rigid Transform1/LConn1
  Rigid Transform1/RConn1 -- F/RConn1
  Rigid Transform/RConn1 -- rev/LConn1
  Rigid Transform/LConn1 -- B/RConn1

== system Out_of_Plane_Model/Chassis, Tires, and Areo/Tire/Rear Tire/Linear Rear Simscape Tire/Simscape/Simscape Multibody Rim&Wheel/Tire_Rim_wth_transient/Roll dof ==
  Bus Creator : BusCreator  Inputs=3
  PS-Simulink Converter : nesl_utility_internal/PS-Simulink Converter  PhysicalDomain=network_engine_domain  SubClassName=ps_output  LeftPortType=input  RightPortType=output  PseudoPeriodic=off  Frequencies=[]  VectorFormat=1-D array  Unit=inherit  AffineConversion=off
  PS-Simulink Converter1 : nesl_utility_internal/PS-Simulink Converter  PhysicalDomain=network_engine_domain  SubClassName=ps_output  LeftPortType=input  RightPortType=output  PseudoPeriodic=off  Frequencies=[]  VectorFormat=1-D array  Unit=inherit  AffineConversion=off
  PS-Simulink Converter2 : nesl_utility_internal/PS-Simulink Converter  PhysicalDomain=network_engine_domain  SubClassName=ps_output  LeftPortType=input  RightPortType=output  PseudoPeriodic=off  Frequencies=[]  VectorFormat=1-D array  Unit=inherit  AffineConversion=off
  Rev : sm_lib/Joints/Revolute Joint  JointMode=Normal  CompositeWrenchDir=FollowerOnBase  CompositeWrenchFrame=BaseFrame  SenseConstraintForce=off  SenseConstraintTorque=off  SenseTotalForce=off  SenseTotalTorque=off  PositionTargetSpecify=off  PositionTargetPriority=High  PositionTargetValue=0  PositionTargetValueUnits=deg  VelocityTargetSpecify=off  VelocityTargetPriority=High  VelocityTargetValue=0  VelocityTargetValueUnits=rad/s  EquilibriumPosition=0  EquilibriumPositionUnits=rad  SpringStiffness=0  SpringStiffnessUnits=N*m/rad  DampingCoefficient=0  DampingCoefficientUnits=N*m/(rad/s)  LowerLimitSpecify=off  LowerLimitBound=-90  LowerLimitBoundUnits=deg  LowerLimitStiffness=1e4  LowerLimitStiffnessUnits=N*m/deg  LowerLimitDamping=10  LowerLimitDampingUnits=N*m/(deg/s)  LowerLimitTransitionRegionWidth=0.1  LowerLimitTransitionRegionWidthUnits=deg  UpperLimitSpecify=off  UpperLimitBound=90  UpperLimitBoundUnits=deg  UpperLimitStiffness=1e4  UpperLimitStiffnessUnits=N*m/deg  UpperLimitDamping=10  UpperLimitDampingUnits=N*m/(deg/s)  UpperLimitTransitionRegionWidth=0.1  UpperLimitTransitionRegionWidthUnits=deg  TorqueActuationMode=NoTorque  MotionActuationMode=ComputedMotion  SensePosition=on  SenseVelocity=on  SenseAcceleration=on  SenseTorqueForce=off  SenseLowerLimitTorqueForce=off  SenseUpperLimitTorqueForce=off
  Unary Minus : UnaryMinus
  Unary Minus1 : UnaryMinus
  Unary Minus2 : UnaryMinus
  Y_-pi/2 : sm_lib/Frames and Transforms/Rigid Transform  RotationMethod=StandardAxis  FollAlignAxisA=+X  BaseAlignAxisA=+Y  FollAlignAxisB=+Y  BaseAlignAxisB=+Z  RotationStandardAxis=+Y  RotationAngle=-pi/2  RotationAngleUnits=rad  RotationArbitraryAxis=[0 0 1]  RotationSequenceAxes=FollowerAxes  RotationSequence=XYX  RotationSequenceAngles=[0 0 0]  RotationSequenceAnglesUnits=deg  RotationMatrix=[1 0 0; 0 1 0; 0 0 1]  Quaternion=[1 0 0 0]  TranslationMethod=None  TranslationCartesianOffset=[0 0 0]  TranslationCartesianOffsetUnits=m  TranslationStandardAxis=+Z  TranslationStandardOffset=0  TranslationStandardOffsetUnits=m  TranslationROffset=0  TranslationROffsetUnits=m  TranslationThetaOffset=0  TranslationThetaOffsetUnits=deg  TranslationZOffset=0  TranslationZOffsetUnits=m
  Y_pi/2 : sm_lib/Frames and Transforms/Rigid Transform  RotationMethod=StandardAxis  FollAlignAxisA=+X  BaseAlignAxisA=+Y  FollAlignAxisB=+Y  BaseAlignAxisB=+Z  RotationStandardAxis=+Y  RotationAngle=pi/2  RotationAngleUnits=rad  RotationArbitraryAxis=[0 0 1]  RotationSequenceAxes=FollowerAxes  RotationSequence=XYX  RotationSequenceAngles=[0 0 0]  RotationSequenceAnglesUnits=deg  RotationMatrix=[1 0 0; 0 1 0; 0 0 1]  Quaternion=[1 0 0 0]  TranslationMethod=None  TranslationCartesianOffset=[0 0 0]  TranslationCartesianOffsetUnits=m  TranslationStandardAxis=+Z  TranslationStandardOffset=0  TranslationStandardOffsetUnits=m  TranslationROffset=0  TranslationROffsetUnits=m  TranslationThetaOffset=0  TranslationThetaOffsetUnits=deg  TranslationZOffset=0  TranslationZOffsetUnits=m
  B : PMIOPort  Side=Left
  F : PMIOPort  Port=2  Side=Right
  A,V,P_WhlRoll : Outport
  wires:
  PS-Simulink Converter/1 -> Unary Minus/1  "WhlPRoll"
  PS-Simulink Converter1/1 -> Unary Minus1/1  "WhlVRoll"
  PS-Simulink Converter2/1 -> Unary Minus2/1  "WhlARoll"
  Bus Creator/1 -> A,V,P_WhlRoll/1  "WhlRrCpX"
  Unary Minus/1 -> Bus Creator/3  "WhlPRoll"
  Unary Minus1/1 -> Bus Creator/2  "WhlVRoll"
  Unary Minus2/1 -> Bus Creator/1  "WhlARoll"
  connections:
  Rev/RConn3 -- PS-Simulink Converter1/LConn1
  PS-Simulink Converter2/LConn1 -- Rev/RConn4
  PS-Simulink Converter/LConn1 -- Rev/RConn2
  Y_-pi/2/RConn1 -- F/RConn1
  Y_pi/2/RConn1 -- Rev/LConn1
  Y_-pi/2/LConn1 -- Rev/RConn1
  Y_pi/2/LConn1 -- B/RConn1

== system Out_of_Plane_Model/Chassis, Tires, and Areo/Tire/Rear Tire/Linear Rear Simscape Tire/Simscape/Simscape Multibody Rim&Wheel/Tire_Rim_wth_transient/dofPitch ==
  HubJoint : sm_lib/Joints/Revolute Joint  JointMode=Normal  CompositeWrenchDir=FollowerOnBase  CompositeWrenchFrame=BaseFrame  SenseConstraintForce=off  SenseConstraintTorque=off  SenseTotalForce=off  SenseTotalTorque=off  PositionTargetSpecify=off  PositionTargetPriority=High  PositionTargetValue=0  PositionTargetValueUnits=deg  VelocityTargetSpecify=on  VelocityTargetPriority=High  VelocityTargetValue=omegao  VelocityTargetValueUnits=rad/s  EquilibriumPosition=0  EquilibriumPositionUnits=deg  SpringStiffness=0  SpringStiffnessUnits=N*m/deg  DampingCoefficient=0  DampingCoefficientUnits=N*m/(rad/s)  LowerLimitSpecify=off  LowerLimitBound=-90  LowerLimitBoundUnits=deg  LowerLimitStiffness=1e4  LowerLimitStiffnessUnits=N*m/deg  LowerLimitDamping=10  LowerLimitDampingUnits=N*m/(deg/s)  LowerLimitTransitionRegionWidth=0.1  LowerLimitTransitionRegionWidthUnits=deg  UpperLimitSpecify=off  UpperLimitBound=90  UpperLimitBoundUnits=deg  UpperLimitStiffness=1e4  UpperLimitStiffnessUnits=N*m/deg  UpperLimitDamping=10  UpperLimitDampingUnits=N*m/(deg/s)  UpperLimitTransitionRegionWidth=0.1  UpperLimitTransitionRegionWidthUnits=deg  TorqueActuationMode=NoTorque  MotionActuationMode=ComputedMotion  SensePosition=off  SenseVelocity=on  SenseAcceleration=on  SenseTorqueForce=off  SenseLowerLimitTorqueForce=off  SenseUpperLimitTorqueForce=off
  PS-Simulink Converter : nesl_utility_internal/PS-Simulink Converter  PhysicalDomain=network_engine_domain  SubClassName=ps_output  LeftPortType=input  RightPortType=output  PseudoPeriodic=off  Frequencies=[]  VectorFormat=1-D array  Unit=inherit  AffineConversion=off
  PS-Simulink Converter1 : nesl_utility_internal/PS-Simulink Converter  PhysicalDomain=network_engine_domain  SubClassName=ps_output  LeftPortType=input  RightPortType=output  PseudoPeriodic=off  Frequencies=[]  VectorFormat=1-D array  Unit=inherit  AffineConversion=off
  Rigid Transform : sm_lib/Frames and Transforms/Rigid Transform  RotationMethod=StandardAxis  FollAlignAxisA=+X  BaseAlignAxisA=+Y  FollAlignAxisB=+Y  BaseAlignAxisB=+Z  RotationStandardAxis=+X  RotationAngle=-pi/2  RotationAngleUnits=rad  RotationArbitraryAxis=[0 0 1]  RotationSequenceAxes=FollowerAxes  RotationSequence=XYX  RotationSequenceAngles=[0 0 0]  RotationSequenceAnglesUnits=deg  RotationMatrix=[1 0 0; 0 1 0; 0 0 1]  Quaternion=[1 0 0 0]  TranslationMethod=None  TranslationCartesianOffset=[0 0 0]  TranslationCartesianOffsetUnits=m  TranslationStandardAxis=+X  TranslationStandardOffset=0  TranslationStandardOffsetUnits=m  TranslationROffset=0  TranslationROffsetUnits=m  TranslationThetaOffset=0  TranslationThetaOffsetUnits=deg  TranslationZOffset=0  TranslationZOffsetUnits=m
  Rigid Transform1 : sm_lib/Frames and Transforms/Rigid Transform  RotationMethod=StandardAxis  FollAlignAxisA=+X  BaseAlignAxisA=+Y  FollAlignAxisB=+Y  BaseAlignAxisB=+Z  RotationStandardAxis=+X  RotationAngle=pi/2  RotationAngleUnits=rad  RotationArbitraryAxis=[0 0 1]  RotationSequenceAxes=FollowerAxes  RotationSequence=XYX  RotationSequenceAngles=[0 0 0]  RotationSequenceAnglesUnits=deg  RotationMatrix=[1 0 0; 0 1 0; 0 0 1]  Quaternion=[1 0 0 0]  TranslationMethod=None  TranslationCartesianOffset=[0 0 0]  TranslationCartesianOffsetUnits=m  TranslationStandardAxis=+X  TranslationStandardOffset=0  TranslationStandardOffsetUnits=m  TranslationROffset=0  TranslationROffsetUnits=m  TranslationThetaOffset=0  TranslationThetaOffsetUnits=deg  TranslationZOffset=0  TranslationZOffsetUnits=m
  B : PMIOPort  Side=Left
  F : PMIOPort  Port=2  Side=Right
  omega : Outport
  omegadot : Outport  Port=2
  wires:
  PS-Simulink Converter/1 -> omega/1
  PS-Simulink Converter1/1 -> omegadot/1
  connections:
  Rigid Transform/LConn1 -- B/RConn1
  Rigid Transform/RConn1 -- HubJoint/LConn1
  Rigid Transform1/RConn1 -- F/RConn1
  HubJoint/RConn1 -- Rigid Transform1/LConn1
  PS-Simulink Converter/LConn1 -- HubJoint/RConn2
  PS-Simulink Converter1/LConn1 -- HubJoint/RConn3

== system Out_of_Plane_Model/Chassis, Tires, and Areo/Tire/Front Tire/Linear Front Simscape Tire/Simscape/Simscape Multibody Rim&Wheel/Tire_Rim_wth_transient/CPSensor/Origin ==
  World Frame : sm_lib/Frames and Transforms/World Frame
  X+pi : sm_lib/Frames and Transforms/Rigid Transform  RotationMethod=StandardAxis  FollAlignAxisA=+X  BaseAlignAxisA=+Y  FollAlignAxisB=+Y  BaseAlignAxisB=+Z  RotationStandardAxis=+X  RotationAngle=pi  RotationAngleUnits=rad  RotationArbitraryAxis=[0 0 1]  RotationSequenceAxes=FollowerAxes  RotationSequence=XYX  RotationSequenceAngles=[0 0 0]  RotationSequenceAnglesUnits=deg  RotationMatrix=[1 0 0; 0 1 0; 0 0 1]  Quaternion=[1 0 0 0]  TranslationMethod=None  TranslationCartesianOffset=[0 0 0]  TranslationCartesianOffsetUnits=m  TranslationStandardAxis=+Z  TranslationStandardOffset=0  TranslationStandardOffsetUnits=m  TranslationROffset=0  TranslationROffsetUnits=m  TranslationThetaOffset=0  TranslationThetaOffsetUnits=deg  TranslationZOffset=0  TranslationZOffsetUnits=m
  F : PMIOPort  Side=Right
  connections:
  X+pi/RConn1 -- F/RConn1
  World Frame/RConn1 -- X+pi/LConn1

== system Out_of_Plane_Model/Chassis, Tires, and Areo/Tire/Rear Tire/Linear Rear Simscape Tire/Simscape/Simscape Multibody Rim&Wheel/Tire_Rim_wth_transient/CPSensor/Origin ==
  World Frame : sm_lib/Frames and Transforms/World Frame
  X+pi : sm_lib/Frames and Transforms/Rigid Transform  RotationMethod=StandardAxis  FollAlignAxisA=+X  BaseAlignAxisA=+Y  FollAlignAxisB=+Y  BaseAlignAxisB=+Z  RotationStandardAxis=+X  RotationAngle=pi  RotationAngleUnits=rad  RotationArbitraryAxis=[0 0 1]  RotationSequenceAxes=FollowerAxes  RotationSequence=XYX  RotationSequenceAngles=[0 0 0]  RotationSequenceAnglesUnits=deg  RotationMatrix=[1 0 0; 0 1 0; 0 0 1]  Quaternion=[1 0 0 0]  TranslationMethod=None  TranslationCartesianOffset=[0 0 0]  TranslationCartesianOffsetUnits=m  TranslationStandardAxis=+Z  TranslationStandardOffset=0  TranslationStandardOffsetUnits=m  TranslationROffset=0  TranslationROffsetUnits=m  TranslationThetaOffset=0  TranslationThetaOffsetUnits=deg  TranslationZOffset=0  TranslationZOffsetUnits=m
  F : PMIOPort  Side=Right
  connections:
  X+pi/RConn1 -- F/RConn1
  World Frame/RConn1 -- X+pi/LConn1
